simulink model "ac_power"  (R2019b)
settings: Solver=VariableStepAuto  StartTime=0.0  StopTime=0.06  MaxStep=0.00001  RelTol=1e-3
model workspace (MAT data in the model file):
  Period = 10
  PhaseDelay = 0
libraries: powerlib x10, powerlib_meascontrol x4, simulink x2
settings Model: Creator=dgander  LastModifiedBy=dgander

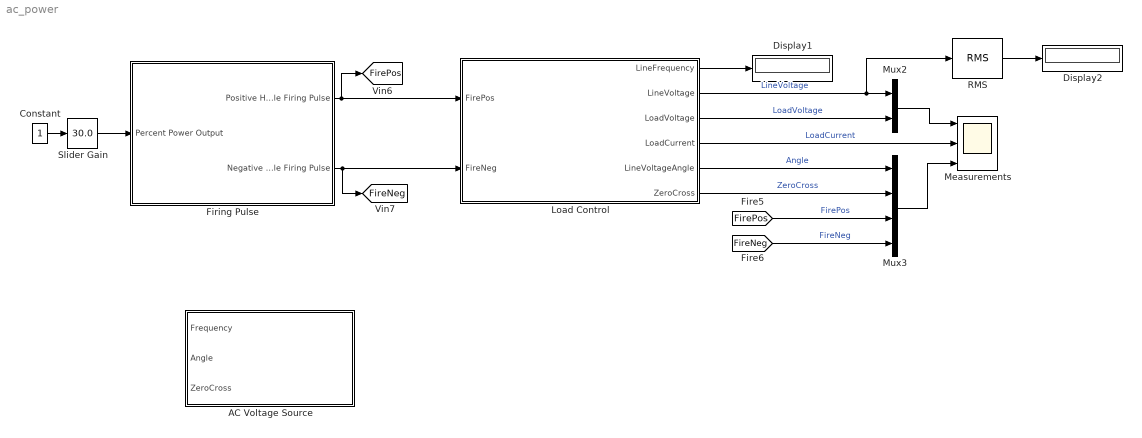
== system ac_power ==
  AC Voltage Source : Subsystem
  Constant : Constant
  Display1 : Display
  Display2 : Display
  Firing Pulse : Subsystem
  Load Control : Subsystem
  Measurements : Scope  NumInputPorts=3
  Mux2 : Mux  Inputs=2
  Mux3 : Mux
  RMS : powerlib_meascontrol/Measurements/RMS  TrueRMS=on  Freq=60  RMSInit=120  Ts=0
      settings: SourceProductName=Simscape Electrical
  Slider Gain : simulink/Math Operations/Slider Gain  gain=30.0  low=0  high=100
  tag scope: FireNeg=global, FirePos=global
  wires:
  Constant/1 -> Slider Gain/1
  Slider Gain/1 -> Firing Pulse/1(Percent Power Output)
  Firing Pulse/1(Positive Half Cycle Firing Pulse) -> Load Control/1(FirePos), [FirePos]
  Firing Pulse/2(Negative Half Cycle Firing Pulse) -> Load Control/2(FireNeg), [FireNeg]
  Mux3/1 -> Measurements/3
  Load Control/6(ZeroCross) -> Mux3/2  "ZeroCross"
  Load Control/5(LineVoltageAngle) -> Mux3/1  "Angle"
  Load Control/4(LoadCurrent) -> Measurements/2  "LoadCurrent"
  Load Control/3(LoadVoltage) -> Mux2/2  "LoadVoltage"
  Load Control/2(LineVoltage) -> RMS/1, Mux2/1  "LineVoltage"
  [FireNeg] -> Mux3/4  "FireNeg"
  [FirePos] -> Mux3/3  "FirePos"
  Mux2/1 -> Measurements/1
  Load Control/1(LineFrequency) -> Display1/1
  RMS/1 -> Display2/1

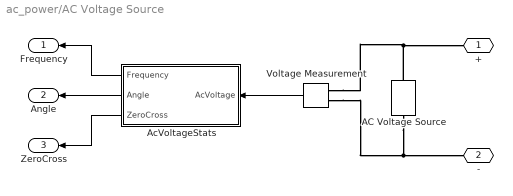
== system ac_power/AC Voltage Source ==
  AC Voltage Source : powerlib/Electrical Sources/AC Voltage Source  Amplitude=120*sqrt(2)  Phase=0  Frequency=60  SampleTime=0  Measurements=None  BusType=swing  Pref=10e3  Qref=0  Qmin=-inf  Qmax=+inf
      settings: SourceProductName=Simscape Electrical
  AcVoltageStats : Subsystem
  Voltage Measurement : powerlib/Measurements/Voltage Measurement  PhasorSimulation=off  OutputType=Complex  PSBequivalent=0
      settings: SourceProductName=Simscape Electrical
  + : PMIOPort  Side=Left
  - : PMIOPort  Port=2  Side=Left
  Frequency : Outport
  Angle : Outport  Port=2
  ZeroCross : Outport  Port=3
  wires:
  Voltage Measurement/1 -> AcVoltageStats/1(AcVoltage)
  AcVoltageStats/3(ZeroCross) -> ZeroCross/1
  AcVoltageStats/1(Frequency) -> Frequency/1
  AcVoltageStats/2(Angle) -> Angle/1
  connections:
  AC Voltage Source/LConn1 -- Voltage Measurement/LConn2 -- -/RConn1
  AC Voltage Source/RConn1 -- Voltage Measurement/LConn1 -- +/RConn1

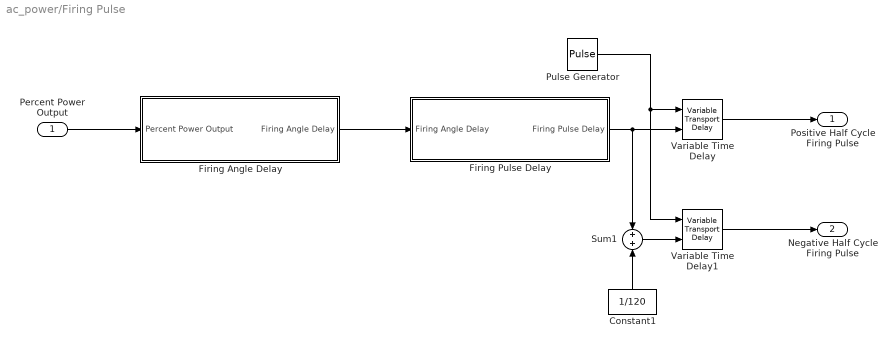
== system ac_power/Firing Pulse ==
  Percent Power Output : Inport
  Constant1 : Constant  Value=1/120
  Firing Angle Delay : Subsystem
  Firing Pulse Delay : Subsystem
  Pulse Generator : DiscretePulseGenerator  PulseType=Time based  Amplitude=6.2  Period=1/60  PulseWidth=5
  Sum1 : Sum
  Variable Time Delay : VariableTransportDelay  MaximumDelay=10  MaximumPoints=7168
  Variable Time Delay1 : VariableTransportDelay  MaximumDelay=10  MaximumPoints=7168
  Positive Half Cycle Firing Pulse : Outport
  Negative Half Cycle Firing Pulse : Outport  Port=2
  wires:
  Variable Time Delay/1 -> Positive Half Cycle Firing Pulse/1
  Pulse Generator/1 -> Variable Time Delay1/1, Variable Time Delay/1
  Firing Angle Delay/1(Firing Angle Delay) -> Firing Pulse Delay/1(Firing Angle Delay)
  Percent Power Output/1 -> Firing Angle Delay/1(Percent Power Output)
  Firing Pulse Delay/1(Firing Pulse Delay) -> Sum1/1, Variable Time Delay/2
  Variable Time Delay1/1 -> Negative Half Cycle Firing Pulse/1
  Sum1/1 -> Variable Time Delay1/2
  Constant1/1 -> Sum1/2

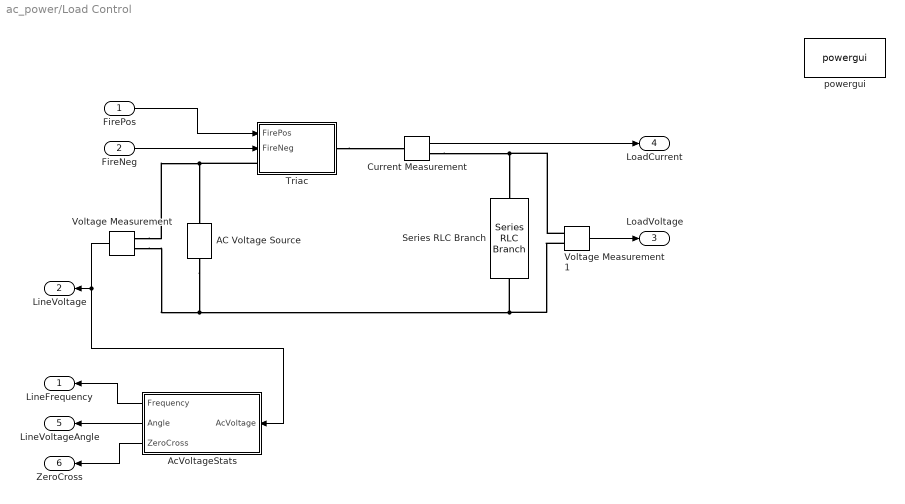
== system ac_power/Load Control ==
  FirePos : Inport
  FireNeg : Inport  Port=2
  AC Voltage Source : powerlib/Electrical Sources/AC Voltage Source  Amplitude=120*sqrt(2)  Phase=0  Frequency=60  SampleTime=0  Measurements=None  BusType=swing  Pref=10e3  Qref=0  Qmin=-inf  Qmax=+inf
      settings: SourceProductName=Simscape Electrical
  AcVoltageStats : Subsystem
  Current Measurement : powerlib/Measurements/Current Measurement  PhasorSimulation=off  OutputType=Complex  PSBequivalent=0
      settings: SourceProductName=Simscape Electrical
  Series RLC Branch : powerlib/Elements/Series RLC Branch  LConnTagsString=__new0  RConnTagsString=__new0  BranchType=R  Resistance=100  Inductance=1e-3  SetiL0=off  InitialCurrent=0  Capacitance=1e-6  Setx0=off  InitialVoltage=0  Measurements=None
      settings: SourceProductName=Simscape Electrical
  Triac : Subsystem
  Voltage Measurement : powerlib/Measurements/Voltage Measurement  PhasorSimulation=off  OutputType=Complex  PSBequivalent=0
      settings: SourceProductName=Simscape Electrical
  Voltage Measurement1 : powerlib/Measurements/Voltage Measurement  PhasorSimulation=off  OutputType=Complex  PSBequivalent=0
      settings: SourceProductName=Simscape Electrical
  powergui : powerlib/powergui  Priority=1  SimulationMode=Continuous  SampleTime=50e-6  frequency=60  Iterations=50  frequencyindice=60  Pbase=100e6  ErrMax=1e-4  UnitsV=kV  UnitsW=MW  buscounter=0  FunctionMessages=off  echomessages=off  EnableUseOfTLC=off  CurrentSourceSwitches=off  DisableSnubberDevices=off  DisableRonSwitches=off  DisableVfSwitches=off  DisplayEquations=off  AutomaticDiscreteSolvers=off  SolverType=Tustin/Backward Euler (TBE)  Interpol=off  ExternalGateDelay=off  methode=off  Ts=100  x0status=blocks  SPID=on  SwTol=0  HookPort=off  NonlinearTolerance=1e-4  nMaxIteration=100  ContinueOnMaxIteration=off  RestoreLinks=warning  ResistiveCurrentMeasurement=off  Frange=[0:2:500]  Ylog=off  Xlog=on  ShowGrid=off  save=off  variable=ZData  structure=0  ZoomFFT=off  StartTime=0.0  cycles=1  DisplayStyle=1  fundamental=60  FreqAxis=off  MaxFrequency=1000  frequencyindicesteady=1  RmsSteady=1  display=off
      settings: SourceProductName=Simscape Electrical
  LineFrequency : Outport
  LineVoltage : Outport  Port=2
  LoadVoltage : Outport  Port=3
  LoadCurrent : Outport  Port=4
  LineVoltageAngle : Outport  Port=5
  ZeroCross : Outport  Port=6
  wires:
  AcVoltageStats/2(Angle) -> LineVoltageAngle/1
  AcVoltageStats/3(ZeroCross) -> ZeroCross/1
  AcVoltageStats/1(Frequency) -> LineFrequency/1
  Current Measurement/1 -> LoadCurrent/1
  Voltage Measurement1/1 -> LoadVoltage/1
  FireNeg/1 -> Triac/2(FireNeg)
  FirePos/1 -> Triac/1(FirePos)
  Voltage Measurement/1 -> AcVoltageStats/1(AcVoltage), LineVoltage/1
  connections:
  AC Voltage Source/LConn1 -- Voltage Measurement/LConn2 -- Series RLC Branch/RConn1 -- Voltage Measurement1/LConn2
  Voltage Measurement/LConn1 -- AC Voltage Source/RConn1 -- Triac/LConn1
  Triac/RConn1 -- Current Measurement/LConn1
  Current Measurement/RConn1 -- Series RLC Branch/LConn1 -- Voltage Measurement1/LConn1

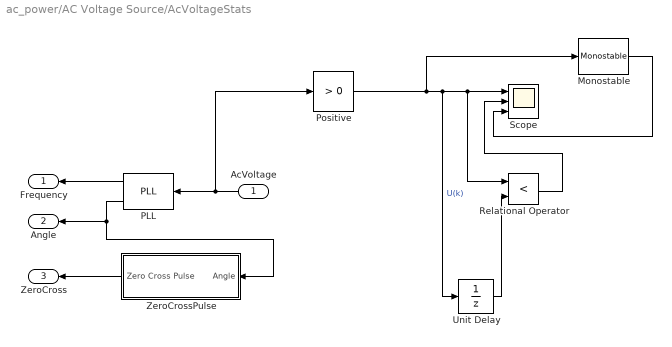
== system ac_power/AC Voltage Source/AcVoltageStats ==
  AcVoltage : Inport
  Monostable : powerlib_meascontrol/Logic/Monostable  EdgeDetect=Rising  PulseDuration=(1/60)*0.05  ic=0  Ts=0
      settings: SourceProductName=Simscape Electrical  SourceProductBaseCode=PS
  PLL : powerlib_meascontrol/PLL/PLL  Fmin=45  Par_Init=[0, 60]  ParK=[180, 3200, 1]  TcD=1e-4  MaxRateChangeFreq=12  FilterCutOffFreq=25  Ts=0  AGC=on
      settings: SourceProductName=Simscape Electrical  SourceProductBaseCode=PS
  Positive : simulink/Logic and Bit Operations/Compare To Zero  relop=>  OutDataTypeStr=uint8
  Relational Operator : RelationalOperator  Operator=<  OutDataTypeStr=boolean  RndMeth=Simplest
  Scope : Scope  NumInputPorts=3
  Unit Delay : UnitDelay  SampleTime=-1  HasFrameUpgradeWarning=on
  ZeroCrossPulse : Subsystem
  Frequency : Outport
  Angle : Outport  Port=2
  ZeroCross : Outport  Port=3
  wires:
  PLL/1 -> Frequency/1
  ZeroCrossPulse/1(Zero Cross Pulse) -> ZeroCross/1
  PLL/2 -> ZeroCrossPulse/1(Angle), Angle/1
  AcVoltage/1 -> Positive/1, PLL/1
  Positive/1 -> Monostable/1, Relational Operator/1, Scope/1, Unit Delay/1  "U(k)"
  Relational Operator/1 -> Scope/2
  Unit Delay/1 -> Relational Operator/2
  Monostable/1 -> Scope/3

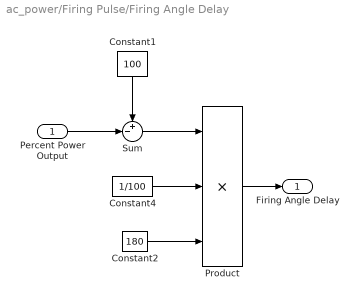
== system ac_power/Firing Pulse/Firing Angle Delay ==
  Percent Power Output : Inport
  Constant1 : Constant  Value=100
  Constant2 : Constant  Value=180
  Constant4 : Constant  Value=1/100
  Product : Product  Inputs=3
  Sum : Sum  Inputs=+-|
  Firing Angle Delay : Outport
  wires:
  Constant4/1 -> Product/2
  Constant2/1 -> Product/3
  Product/1 -> Firing Angle Delay/1
  Percent Power Output/1 -> Sum/2
  Sum/1 -> Product/1
  Constant1/1 -> Sum/1

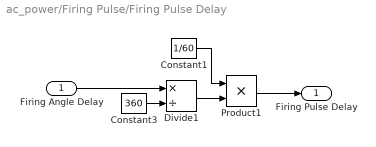
== system ac_power/Firing Pulse/Firing Pulse Delay ==
  Firing Angle Delay : Inport
  Constant1 : Constant  Value=1/60
  Constant3 : Constant  Value=360
  Divide1 : Product  Inputs=*/
  Product1 : Product
  Firing Pulse Delay : Outport
  wires:
  Product1/1 -> Firing Pulse Delay/1
  Firing Angle Delay/1 -> Divide1/1
  Constant1/1 -> Product1/1
  Divide1/1 -> Product1/2
  Constant3/1 -> Divide1/2

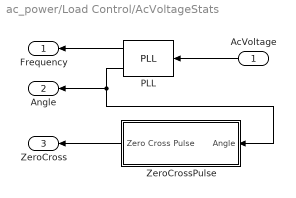
== system ac_power/Load Control/AcVoltageStats ==
  AcVoltage : Inport
  PLL : powerlib_meascontrol/PLL/PLL  Fmin=45  Par_Init=[0, 60]  ParK=[180, 3200, 1]  TcD=1e-4  MaxRateChangeFreq=12  FilterCutOffFreq=25  Ts=0  AGC=on
      settings: SourceProductName=Simscape Electrical  SourceProductBaseCode=PS
  ZeroCrossPulse : Subsystem
  Frequency : Outport
  Angle : Outport  Port=2
  ZeroCross : Outport  Port=3
  wires:
  PLL/1 -> Frequency/1
  ZeroCrossPulse/1(Zero Cross Pulse) -> ZeroCross/1
  PLL/2 -> Angle/1, ZeroCrossPulse/1(Angle)
  AcVoltage/1 -> PLL/1

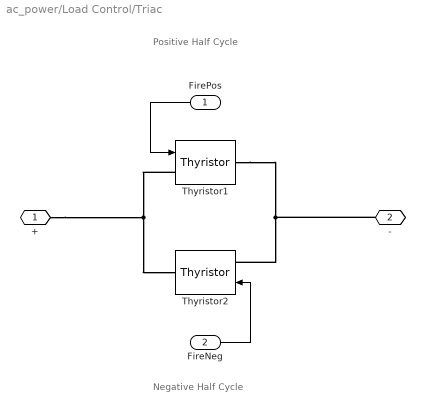
== system ac_power/Load Control/Triac ==
  note: Positive Half Cycle
  note: Negative Half Cycle
  FirePos : Inport
  FireNeg : Inport  Port=2
  Thyristor1 : powerlib/Power Electronics/Thyristor  Ron=0.001  Lon=0  Vf=0.8  IC=0  Rs=500  Cs=250e-9  Measurements=off
      settings: SourceProductName=Simscape Electrical
  Thyristor2 : powerlib/Power Electronics/Thyristor  Ron=0.001  Lon=0  Vf=0.8  IC=0  Rs=500  Cs=250e-9  Measurements=off
      settings: SourceProductName=Simscape Electrical
  + : PMIOPort  Side=Left
  - : PMIOPort  Port=2  Side=Right
  wires:
  FirePos/1 -> Thyristor1/1
  FireNeg/1 -> Thyristor2/1
  connections:
  Thyristor1/LConn1 -- +/RConn1 -- Thyristor2/RConn1
  Thyristor1/RConn1 -- -/RConn1 -- Thyristor2/LConn1

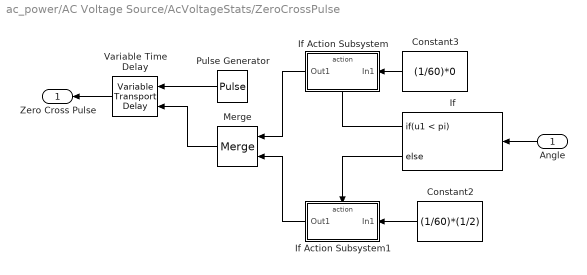
== system ac_power/AC Voltage Source/AcVoltageStats/ZeroCrossPulse ==
  Angle : Inport
  Constant2 : Constant  Value=(1/60)*(1/2)
  Constant3 : Constant  Value=(1/60)*0
  If : If  IfExpression=u1 < pi
  If Action Subsystem : Subsystem  TreatAsAtomicUnit=on
  If Action Subsystem1 : Subsystem  TreatAsAtomicUnit=on
  Merge : Merge
  Pulse Generator : DiscretePulseGenerator  PulseType=Time based  Amplitude=6.2  Period=1/60  PulseWidth=5
  Variable Time Delay : VariableTransportDelay  MaximumDelay=10  MaximumPoints=7168  ZeroDelay=on
  Zero Cross Pulse : Outport
  wires:
  Pulse Generator/1 -> Variable Time Delay/1
  Constant3/1 -> If Action Subsystem/1(In1)
  Constant2/1 -> If Action Subsystem1/1(In1)
  Merge/1 -> Variable Time Delay/2
  If/1 -> If Action Subsystem/Action
  If/2 -> If Action Subsystem1/Action
  Variable Time Delay/1 -> Zero Cross Pulse/1
  Angle/1 -> If/1
  If Action Subsystem/1(Out1) -> Merge/1
  If Action Subsystem1/1(Out1) -> Merge/2

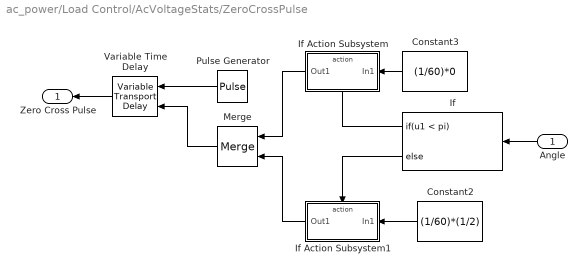
== system ac_power/Load Control/AcVoltageStats/ZeroCrossPulse ==
  Angle : Inport
  Constant2 : Constant  Value=(1/60)*(1/2)
  Constant3 : Constant  Value=(1/60)*0
  If : If  IfExpression=u1 < pi
  If Action Subsystem : Subsystem  TreatAsAtomicUnit=on
  If Action Subsystem1 : Subsystem  TreatAsAtomicUnit=on
  Merge : Merge
  Pulse Generator : DiscretePulseGenerator  PulseType=Time based  Amplitude=6.2  Period=1/60  PulseWidth=5
  Variable Time Delay : VariableTransportDelay  MaximumDelay=10  MaximumPoints=7168  ZeroDelay=on
  Zero Cross Pulse : Outport
  wires:
  Pulse Generator/1 -> Variable Time Delay/1
  Constant3/1 -> If Action Subsystem/1(In1)
  Constant2/1 -> If Action Subsystem1/1(In1)
  Merge/1 -> Variable Time Delay/2
  If/1 -> If Action Subsystem/Action
  If/2 -> If Action Subsystem1/Action
  Variable Time Delay/1 -> Zero Cross Pulse/1
  Angle/1 -> If/1
  If Action Subsystem/1(Out1) -> Merge/1
  If Action Subsystem1/1(Out1) -> Merge/2

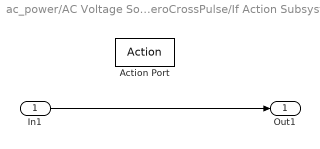
== system ac_power/AC Voltage Source/AcVoltageStats/ZeroCrossPulse/If Action Subsystem ==
  In1 : Inport
  Action Port : ActionPort  ActionPortLabel=if(u1 < pi)
  Out1 : Outport
  wires:
  In1/1 -> Out1/1

== system ac_power/AC Voltage Source/AcVoltageStats/ZeroCrossPulse/If Action Subsystem1 ==
  In1 : Inport
  Action Port : ActionPort  ActionPortLabel=else
  Out1 : Outport
  wires:
  In1/1 -> Out1/1

== system ac_power/Load Control/AcVoltageStats/ZeroCrossPulse/If Action Subsystem ==
  In1 : Inport
  Action Port : ActionPort  ActionPortLabel=if(u1 < pi)
  Out1 : Outport
  wires:
  In1/1 -> Out1/1

== system ac_power/Load Control/AcVoltageStats/ZeroCrossPulse/If Action Subsystem1 ==
  In1 : Inport
  Action Port : ActionPort  ActionPortLabel=else
  Out1 : Outport
  wires:
  In1/1 -> Out1/1
